simulink model "StanfordArmModel_backcompatible"  (R2017a)
settings: Solver=FixedStepAuto  StartTime=0.0  StopTime=inf  RelTol=1e-3
libraries: simulink x8
settings Model: Creator=crbon  LastModifiedBy=Chris
settings DataIOCC: ReturnWorkspaceOutputs=on
settings SFSimCC: SimUseLocalCustomCode=on
settings RTWCC: RTWUseLocalCustomCode=on

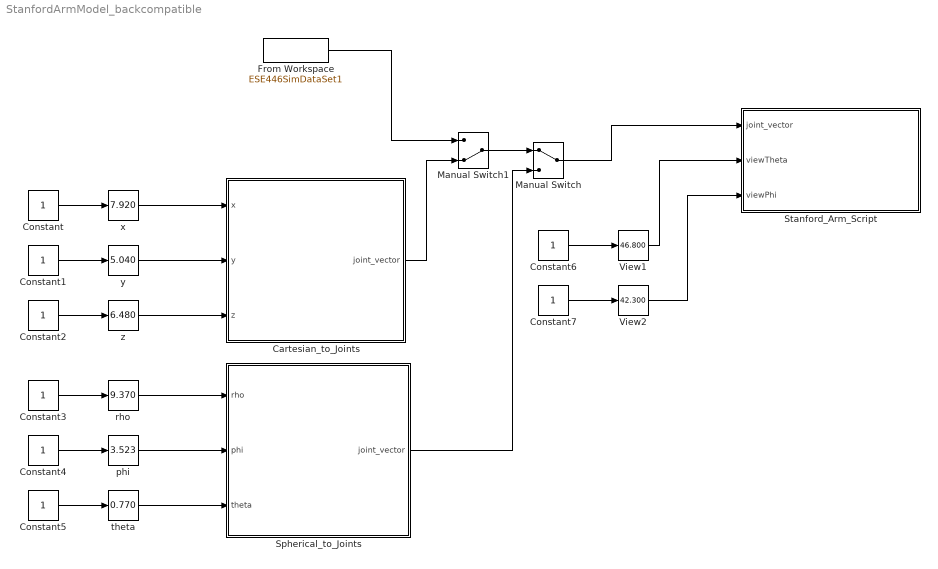
== system StanfordArmModel_backcompatible ==
  Cartesian_to_Joints : MATLAB Function  TreatAsAtomicUnit=on
  Constant{,1..7} (8 alike) : Constant
  From Workspace : FromWorkspace  VariableName=ESE446SimDataSet1  SampleTime=.01
  Manual Switch : ManualSwitch
  Manual Switch1 : ManualSwitch  CurrentSetting=0
  Spherical_to_Joints : MATLAB Function  TreatAsAtomicUnit=on
  Stanford_Arm_Script : MATLAB Function  TreatAsAtomicUnit=on
  View1 : simulink/Math Operations/Slider Gain  gain=46.800  low=0  high=90
  View2 : simulink/Math Operations/Slider Gain  gain=42.300  low=0  high=90
  phi : simulink/Math Operations/Slider Gain  gain=3.523  low=0  high=6.18
  "rho " : simulink/Math Operations/Slider Gain  gain=9.370  low=3  high=10
  theta : simulink/Math Operations/Slider Gain  gain=0.770  low=.25  high=2.85
  x : simulink/Math Operations/Slider Gain  gain=7.920  low=-12  high=12
  y : simulink/Math Operations/Slider Gain  gain=5.040  low=-12  high=12
  z : simulink/Math Operations/Slider Gain  gain=6.480  low=-12  high=12
  wires:
  Manual Switch/1 -> Stanford_Arm_Script/1(joint_vector)
  Manual Switch1/1 -> Manual Switch/1
  Constant/1 -> x/1
  Constant1/1 -> y/1
  Constant2/1 -> z/1
  Constant5/1 -> theta/1
  Constant4/1 -> phi/1
  Constant3/1 -> "rho "/1
  x/1 -> Cartesian_to_Joints/1(x)
  y/1 -> Cartesian_to_Joints/2(y)
  z/1 -> Cartesian_to_Joints/3(z)
  "rho "/1 -> Spherical_to_Joints/1(rho)
  phi/1 -> Spherical_to_Joints/2(phi)
  theta/1 -> Spherical_to_Joints/3(theta)
  Cartesian_to_Joints/1(joint_vector) -> Manual Switch1/2
  Spherical_to_Joints/1(joint_vector) -> Manual Switch/2
  View2/1 -> Stanford_Arm_Script/3(viewPhi)
  View1/1 -> Stanford_Arm_Script/2(viewTheta)
  Constant7/1 -> View2/1
  Constant6/1 -> View1/1
  From Workspace/1 -> Manual Switch1/1

== matlab function StanfordArmModel_backcompatible/Cartesian_to_Joints ==
  data: x input; y input; z input; joint_vector output
% creates a joint vector for the position of the stanford arm from 
% a cartesian input; doesn't calculate wrist angles or EOAT
function joint_vector  = Cartesian_to_Joints(x,y,z)
%% initialize
joint_vector = zeros(1,6);

%% Calculate spherical
phi = atan2(y,x);
rho = sqrt(x.^2 + y.^2 + z.^2);
theta = acos(z/rho);

%% d3 
d3 = sqrt(rho^2-4);
joint_vector(3) = d3;

%% theta2
theta2 = acos(rho*cos(theta)/d3);
joint_vector(2) = theta2;

%% theta1
alpha = atan2(2,d3*sin(theta2));

theta1 = phi - alpha;
joint_vector(1) = theta1;
end

== matlab function StanfordArmModel_backcompatible/Stanford_Arm_Script ==
  data: joint_vector input; viewTheta input; viewPhi input
function Stanford_Arm_Script(joint_vector, viewTheta, viewPhi)

%% Unpack Joint Vector
theta1 = joint_vector(1);
theta2 = joint_vector(2);
d3     = joint_vector(3);
theta4 = joint_vector(4);
theta5 = joint_vector(5)+pi/2;
theta6 = joint_vector(6);

%% Calculate endpoints for visualization
% Cartesian
x = cos(theta1)*d3*sin(theta2)-sin(theta1)*2;
y = sin(theta1)*d3*sin(theta2)+cos(theta1)*2;
z = d3*cos(theta2);

% Spherical
Rho = sqrt(d3^2+4);
% Max elevation for current value of d3
phi_max = atan(d3/2);
% create surface spherical shell for current d3
Phi_grid=linspace(-phi_max,phi_max);
Theta_grid=linspace(0,2*pi);
[Phi_grid,Theta_grid]=meshgrid(Phi_grid,Theta_grid);
[X,Y,Z]=sph2cart(Theta_grid,Phi_grid,Rho);


%% Define Links/ Robot Shapes
origin = [0;0;0];

Base  = [...
         -1  -1  -1  -1  -1   1   1  -1   1   1  -1   1   1  -1   1   1;...
          1  -1  -1   1   1   1   1   1   1  -1  -1  -1  -1  -1  -1   1;...
        -15 -15  -1  -1 -15 -15  -1  -1  -1  -1  -1  -1 -15 -15 -15 -15;...
];

Link1 = [...
          1  -1  -1   1   1   1   1   1   1  -1  -1  -1  -1  -1  -1   1;...
          1   1  -1  -1   1   1  -1  -1  -1  -1  -1  -1   1   1   1   1;...
         -1  -1  -1  -1  -1   1   1  -1   1   1  -1   1   1  -1   1   1;...
];

Link2 = [...
          1  -1  -1   1   1   1   1   1   1  -1  -1  -1  -1  -1  -1   1;...
          1   1  -1  -1   1   1  -1  -1  -1  -1  -1  -1   1   1   1   1;...
         -1  -1  -1  -1  -1   1   1  -1   1   1  -1   1   1  -1   1   1;...
];

%no visible link in model
Link3 = [0;0;0];

Link4 = [...
        -.5 -.5 -.5 -.5 -.5  .5  .5 -.5  .5  .5 -.5  .5  .5 -.5  .5  .5;...
         .5 -.5 -.5  .5  .5  .5  .5  .5  .5 -.5 -.5 -.5 -.5 -.5 -.5  .5;...
        -15 -15  -1  -1 -15 -15  -1  -1  -1  -1  -1  -1 -15 -15 -15 -15;...
];

Link5 = [...
          1  -1  -1   1   1   1   1   1   1  -1  -1  -1  -1  -1  -1   1;...
          1   1  -1  -1   1   1  -1  -1  -1  -1  -1  -1   1   1   1   1;...
         -1  -1  -1  -1  -1   1   1  -1   1   1  -1   1   1  -1   1   1;...
];

Link6 = [...
        -.5 -.5 -.5 -.5 -.5  .5  .5 -.5  .5  .5 -.5  .5  .5 -.5  .5  .5;...
         .5 -.5 -.5  .5  .5  .5  .5  .5  .5 -.5 -.5 -.5 -.5 -.5 -.5  .5;...
          5   5   1   1   5   5   1   1   1   1   1   1   5   5   5   5;...
];

% shape of axis figure for base and EOAT
axes  = [...
         0 1.5 0  0  0  0  0;...
         0  0  0 1.5 0  0  0;...
         0  0  0  0  0 1.5 0;...
];

%% Transform Link 1
BaseLink1= TRANS01SF(Link1 ,theta1);

%% Transform Link 2
Link12   = TRANS12SF(Link2 ,theta2);
BaseLink2= TRANS01SF(Link12,theta1);
BaseLink2O = TRANS01SF(TRANS12SF(origin,theta2),theta1);

%% Transform Link 3
%no visible links
%   Link23   = TRANS23SF(Link3 ,d3    );
%   Link13   = TRANS12SF(Link23,theta2);
%   BaseLink3= TRANS01SF(Link13,theta1);
BaseLink3O = TRANS01SF(TRANS12SF(TRANS23SF(origin,d3),theta2),theta1);

%% Transform Link 4
Link34   = TRANS34SF(Link4 ,theta4);
Link24   = TRANS23SF(Link34,d3    );
Link14   = TRANS12SF(Link24,theta2);
BaseLink4= TRANS01SF(Link14,theta1);

%% Transform Link 5
Link45   = TRANS45SF(Link5 ,theta5);
Link35   = TRANS34SF(Link45,theta4);
Link25   = TRANS23SF(Link35,d3    );
Link15   = TRANS12SF(Link25,theta2);
BaseLink5= TRANS01SF(Link15,theta1);

%% Transform Link 6
Link56   = TRANS56SF(Link6 ,theta6);
Link46   = TRANS45SF(Link56,theta5);
Link36   = TRANS34SF(Link46,theta4);
Link26   = TRANS23SF(Link36,d3    );
Link16   = TRANS12SF(Link26,theta2);
BaseLink6= TRANS01SF(Link16,theta1);

%% Transform EOAT
Link67   = TRANS67SF(axes         );
Link57   = TRANS56SF(Link67,theta6);
Link47   = TRANS45SF(Link57,theta5);
Link37   = TRANS34SF(Link47,theta4);
Link27   = TRANS23SF(Link37,d3    );
Link17   = TRANS12SF(Link27,theta2);
BaseEOAT = TRANS01SF(Link17,theta1);


%% Plotting
plot3(Base(1,:),Base(2,:),Base(3,:),'k-')
axis([-15 15 -15 15 -15 15]);
grid on
hold on
plot3(BaseLink1(1,:),BaseLink1(2,:),BaseLink1(3,:),'b-', 'LineWidth', 2)
plot3(BaseLink2(1,:),BaseLink2(2,:),BaseLink2(3,:),'g-', 'LineWidth', 2)
%   plot3(BaseLink3(1,:),BaseLink3(2,:),BaseLink3(3,:),'k-', 'LineWidth', 2)
plot3(BaseLink4(1,:),BaseLink4(2,:),BaseLink4(3,:),'m-', 'LineWidth', 2)
plot3(BaseLink5(1,:),BaseLink5(2,:),BaseLink5(3,:),'b-', 'LineWidth', 2)
% plot3(BaseLink6(1,:),BaseLink6(2,:),BaseLink6(3,:),'k-', 'LineWidth', 2)
plot3(BaseLink2O(1,:),BaseLink2O(2,:),BaseLink2O(3,:),'r*', 'LineWidth', 2)
plot3(BaseLink3O(1,:),BaseLink3O(2,:),BaseLink3O(3,:),'r*', 'LineWidth', 2)
plot3(axes(1,:),   axes(2,:),   axes(3,:),   'r-', 'LineWidth', 2)
plot3(axes(1,1),   axes(2,1),   axes(3,1),   'r*', 'LineWidth', 2)
% plot3(BaseEOAT(1,:), BaseEOAT(2,:), BaseEOAT(3,:), 'r-', 'LineWidth', 2)
% plot3(BaseEOAT(1,1), BaseEOAT(2,1), BaseEOAT(3,1), 'r*', 'LineWidth', 2)
surf(X,Y,Z, 'EdgeColor', 'none');
alpha 0.2
% draws line to wrist
plot3([0 x],[0 y],[0 z],'k-', 'LineWidth',4)
xlabel('X');
ylabel('Y');
zlabel('Z');
view(viewTheta,viewPhi);
hold off

end

== matlab function StanfordArmModel_backcompatible/Spherical_to_Joints ==
  data: rho input; phi input; theta input; joint_vector output
% creates a joint vector for the position of the stanford arm from 
% a spherical input; doesn't calculate wrist angles or EOAT
function joint_vector  = Spherical_to_Joints(rho,phi,theta)
%% initialize
joint_vector = zeros(1,6);

%% d3
d3 = sqrt(rho^2-4);
joint_vector(3) = d3;

%% theta2
theta2 = acos(rho*cos(theta)/d3);
joint_vector(2) = theta2;

%% theta1
alpha = atan2(2,d3*sin(theta2));

theta1 = phi - alpha;
joint_vector(1) = theta1;
end
